simulink model "CryoDet6"  (R2015a)
settings: Solver=ode45  SolverMode=SingleTasking  StartTime=0.0  StopTime=1e-3  MaxStep=Tclk/8  RelTol=1e-3
values from neighbouring files (symbols this model uses):
  Fclk = Fadc/2    (= 185000000)    [setupCryoFPGA.m]    (also in setupCryoNew.m)
  noise = exp(1i*phi)    [setupCryoFPGA.m]    (also in setupCryoNew.m = exp(2i*pi*rand(1, noiseLen)))
  noiseLen = 128    [setupCryoFPGA.m]    (also in setupCryoNew.m)
  noiseSteps = 32    [setupCryoFPGA.m]    (also in setupCryoNew.m)
  notch = tf( [1 a*wNotch/Q wNotch^2], [1 wNotch/Q wNotch^2])    [setupCryoFPGA.m]    (also in setupCryoNew.m)
  notch2 = tf( [1 a*wNotch/Q wNotch^2], [1 wNotch/Q wNotch^2])    [setupCryoFPGA.m]    (also in setupCryoNew.m)
  setupVers = 5    [setupCryoFPGA.m]    (also in setupCryoNew.m = 21)
  Tclk = 1/Fclk    (= 5.40540540541e-09)    [setupCryoFPGA.m]    (also in setupCryoNew.m)
  wTs1 = w1*Ts1    (= 0.0271705310581)    [setupCryoFPGA.m]
undefined symbols (not defined in the file or in its folder): AXI4, Lite, xlipgetpartsetting
libraries: xbsIndex_r4 x516, simulink x1
(part 1 of 6)
settings Model: CovSFcnEnable=off  Creator=ssmith  LastModifiedBy=ssmith
settings OptimizationCC: BlockReduction=off  BooleanDataType=off
settings DebuggingCC: SaveWithParameterizedLinksMsg=none  UnderspecifiedInitializationDetection=Classic  MergeDetectMultiDrivingBlocksExec=none  SignalResolutionControl=TryResolveAllWithWarning
settings HardwareCC: TargetUnknown=on

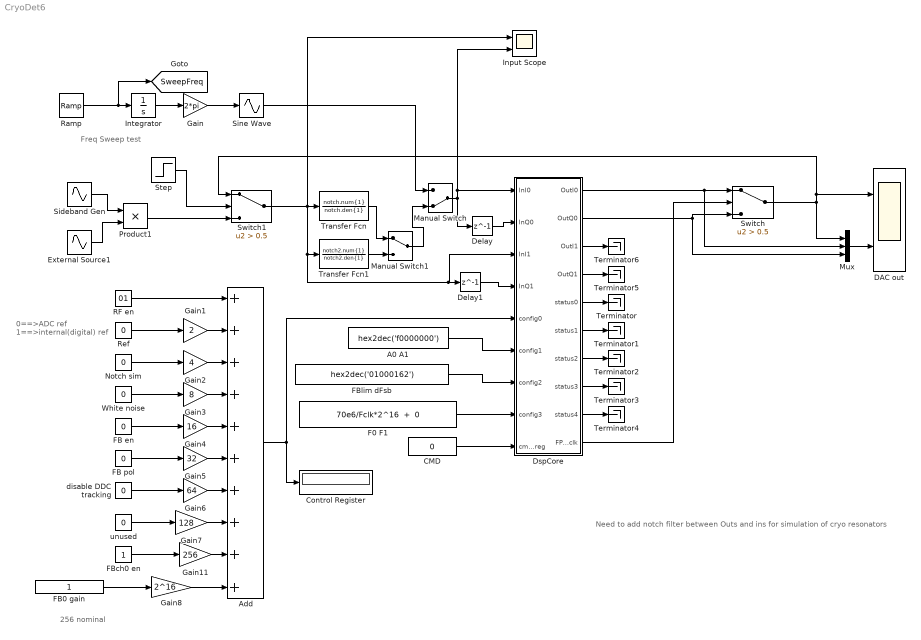
== system CryoDet6 ==
  note: 256 nominal
  note: 0==>ADC ref
      | 1==>internal(digital) ref
  note: Freq Sweep test
  note: Need to add notch filter between Outs and ins for simulation of cryo resonators
  A0 A1 : Constant  Value=hex2dec('f0000000')  SampleTime=Tclk
  Add : Sum  Inputs=++++++++++
  CMD : Constant  Value=0  SampleTime=Tclk
  Control Register : Display
      settings: Format=hex (Stored Integer)  Decimation=1000
  DAC out : Scope  NumInputPorts=2
      settings: TickLabels=on  TimeRange=3.316216230427035e-06  YMin=-1~-1  YMax=1~1  SaveName=DACscope  SampleTime=0.1e-6
  Delay : Delay  DelayLength=1  SampleTime=Tclk/2
  Delay1 : Delay  DelayLength=1  SampleTime=Tclk/2
  DspCore : Subsystem
  External Source1 : Sin  Amplitude=.8  Frequency=2*pi*70e6  SampleTime=0
  F0 F1 : Constant  Value="70e6/Fclk*2^16  +  0"  SampleTime=Tclk
  FB en : Constant  Value=0  SampleTime=Tclk
  FB pol : Constant  Value=0  SampleTime=Tclk
  FB0 gain : Constant  SampleTime=Tclk
  FBch0 en : Constant  SampleTime=Tclk
  FBlim dFsb : Constant  Value=hex2dec('01000162')  SampleTime=Tclk
  Gain : Gain  Gain=2*pi
  Gain1 : Gain  Gain=2
  Gain11 : Gain  Gain=256
  Gain2 : Gain  Gain=4
  Gain3 : Gain  Gain=8
  Gain4 : Gain  Gain=16
  Gain5 : Gain  Gain=32
  Gain6 : Gain  Gain=64
  Gain7 : Gain  Gain=128
  Gain8 : Gain  Gain=2^16
  Input Scope : Scope  NumInputPorts=2
      settings: TimeRange=6.755405405405412e-06  YMin=-1~-5e-147  YMax=1~5e-147  SaveName=ScopeData18
  Integrator : Integrator
  Manual Switch : ManualSwitch  CurrentSetting=0
  Manual Switch1 : ManualSwitch
  Mux : Mux  Inputs=3
  Notch sim : Constant  Value=0  SampleTime=Tclk
  Product1 : Product
  RF en : Constant  Value=01  SampleTime=Tclk
  Ramp : simulink/Sources/Ramp  slope=0.4e6/1e-3  start=0  X0=69.8e6
  Ref : Constant  Value=0  SampleTime=Tclk
  Sideband Gen : Sin  Amplitude=0.18  Bias=0.8  Frequency=2*pi*1e6  SampleTime=0
  Sine Wave : Sin  TimeSource=Use external signal  SampleTime=0
  Step : Step  Time=1e-6  SampleTime=0
  Switch : Switch  Criteria=u2 > Threshold  Threshold=0.5
  Switch1 : Switch  Criteria=u2 > Threshold  Threshold=0.5
  Terminator{,1..6} (7 alike) : Terminator
  Transfer Fcn : TransferFcn  Numerator=notch.num{1}  Denominator=notch.den{1}
  Transfer Fcn1 : TransferFcn  Numerator=notch2.num{1}  Denominator=notch2.den{1}
  White noise : Constant  Value=0  SampleTime=Tclk
  disable DDC tracking : Constant  Value=0  SampleTime=Tclk
  unused : Constant  Value=0  SampleTime=Tclk
  tag scope: SweepFreq=global
  wires:
  Add/1 -> DspCore/5(config0), Control Register/1
  A0 A1/1 -> DspCore/6(config1)
  FBlim dFsb/1 -> DspCore/7(config2)
  F0 F1/1 -> DspCore/8(config3)
  CMD/1 -> DspCore/9(cmd_reg)
  Delay/1 -> DspCore/2(InQ0)
  Delay1/1 -> DspCore/4(InQ1)
  DspCore/5(status0) -> Terminator/1
  DspCore/6(status1) -> Terminator1/1
  DspCore/7(status2) -> Terminator2/1
  DspCore/8(status3) -> Terminator3/1
  DspCore/9(status4) -> Terminator4/1
  Sideband Gen/1 -> Product1/1
  DspCore/10(FPGAclk) -> Switch/2
  DspCore/2(OutQ0) -> Mux/3, Switch/3
  Switch/1 -> DAC out/1, Switch1/1, Mux/1
  DspCore/1(OutI0) -> Switch/1, Mux/2
  Product1/1 -> Switch1/3
  Step/1 -> Switch1/2
  Manual Switch/1 -> Input Scope/2, DspCore/1(InI0), Delay/1
  Sine Wave/1 -> Manual Switch/1
  Ramp/1 -> [SweepFreq], Integrator/1
  Gain/1 -> Sine Wave/1
  Integrator/1 -> Gain/1
  Switch1/1 -> Transfer Fcn1/1, DspCore/3(InI1), Delay1/1, Input Scope/1, Transfer Fcn/1
  External Source1/1 -> Product1/2
  Transfer Fcn1/1 -> Manual Switch1/2
  Transfer Fcn/1 -> Manual Switch1/1
  Manual Switch1/1 -> Manual Switch/2
  RF en/1 -> Add/1
  Ref/1 -> Gain1/1
  Notch sim/1 -> Gain2/1
  White noise/1 -> Gain3/1
  FB en/1 -> Gain4/1
  FB pol/1 -> Gain5/1
  disable DDC tracking/1 -> Gain6/1
  unused/1 -> Gain7/1
  Gain1/1 -> Add/2
  Gain2/1 -> Add/3
  Gain3/1 -> Add/4
  Gain4/1 -> Add/5
  Gain5/1 -> Add/6
  Gain6/1 -> Add/7
  Gain7/1 -> Add/8
  FBch0 en/1 -> Gain11/1
  Gain11/1 -> Add/9
  Gain8/1 -> Add/10
  FB0 gain/1 -> Gain8/1
  DspCore/3(OutI1) -> Terminator6/1
  DspCore/4(OutQ1) -> Terminator5/1
  Mux/1 -> DAC out/2

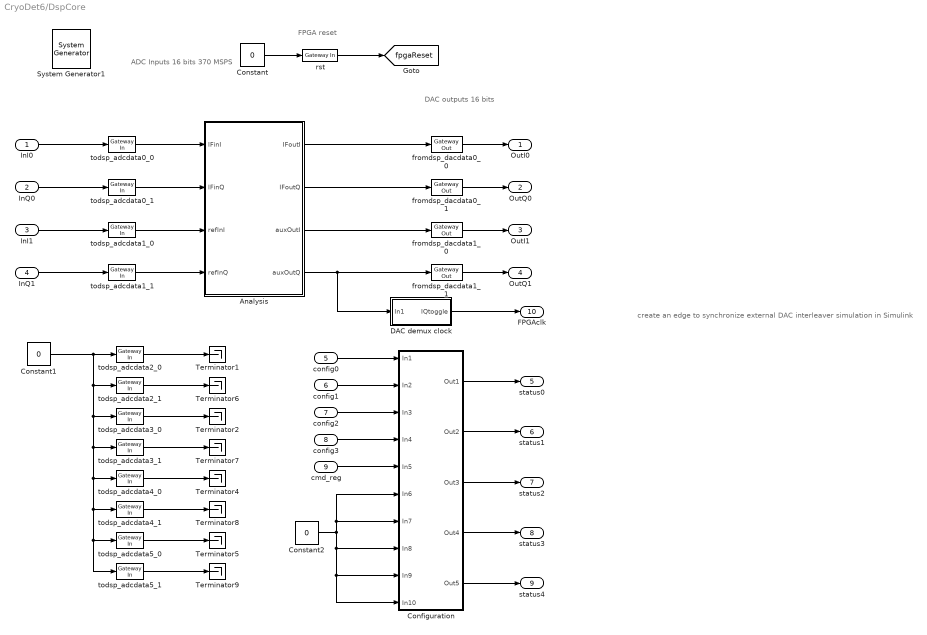
== system CryoDet6/DspCore ==
  note: create an edge to synchronize external DAC interleaver simulation in Simulink
  note: DAC outputs
      | 16 bits
  note: ADC Inputs
      | 16 bits
      | 370 MSPS
  note: FPGA reset
  InI0 : Inport
  InQ0 : Inport  Port=2
  InI1 : Inport  Port=3
  InQ1 : Inport  Port=4
  config0 : Inport  Port=5
  config1 : Inport  Port=6
  config2 : Inport  Port=7
  config3 : Inport  Port=8
  cmd_reg : Inport  Port=9
  " System Generator1" : xbsIndex_r4/ System Generator  Tag=genX  xilinxfamily=kintexu  part=xcku040  speed=-2-e  package=ffva1156  synthesis_tool=Vivado  clock_wrapper=Clock Enables  directory=./netlist  proj_type=Vivado  Synth_file=Vivado Synthesis Defaults  Impl_file=Vivado Implementation Defaults  testbench=off  simulink_period=Tclk  sysclk_period=Tclk*1e9  dcm_input_clock_period=10  incr_netlist=off  trim_vbits=Everywhere in SubSystem  dbl_ovrd=According to Block Masks  core_generation=According to Block Masks  run_coregen=off  deprecated_control=off  eval_field=0  block_type=sysgen
  Analysis : Subsystem
  Configuration : Subsystem
  Constant : Constant  Value=0
  Constant1 : Constant  Value=0
  Constant2 : Constant  Value=0
  DAC demux clock : Subsystem
  Terminator{1..2,4..9} (8 alike) : Terminator
  fromdsp_dacdata0_0 : xbsIndex_r4/Gateway Out  inherit_from_input=on  hdl_port=on  rows=1  columns=1  UseAsDAC=off  DACChannel='1'  interface=None  automatic_assignment=on  address_offset=hex2dec('00')  intf_name=''  intf_description=''  timing_constraint=None  locs_specified=off  LOCs={}  io_standard={}  block_type=gatewayout
  fromdsp_dacdata0_1 : xbsIndex_r4/Gateway Out  inherit_from_input=on  hdl_port=on  rows=1  columns=1  UseAsDAC=off  DACChannel='1'  interface=None  automatic_assignment=on  address_offset=hex2dec('00')  intf_name=''  intf_description=''  timing_constraint=None  locs_specified=off  LOCs={}  io_standard={}  block_type=gatewayout
  fromdsp_dacdata1_0 : xbsIndex_r4/Gateway Out  inherit_from_input=on  hdl_port=on  rows=1  columns=1  UseAsDAC=off  DACChannel='1'  interface=None  automatic_assignment=on  address_offset=hex2dec('00')  intf_name=''  intf_description=''  timing_constraint=None  locs_specified=off  LOCs={}  io_standard={}  block_type=gatewayout
  fromdsp_dacdata1_1 : xbsIndex_r4/Gateway Out  inherit_from_input=off  hdl_port=on  rows=1  columns=1  UseAsDAC=off  DACChannel='1'  interface=None  automatic_assignment=on  address_offset=hex2dec('00')  intf_name=''  intf_description=''  timing_constraint=None  locs_specified=off  LOCs={}  io_standard={}  block_type=gatewayout
  rst : xbsIndex_r4/Gateway In  gui_display_data_type=Boolean  arith_type=Boolean  n_bits=16  bin_pt=14  preci_type=Single  exp_width=8  frac_width=24  rows=1  columns=1  quantization="Round  (unbiased: +/- Inf)"  overflow=Saturate  period=Tclk  UseAsADC=off  ADCChannel='1'  interface=None  automatic_assignment=on  address_offset=hex2dec('00')  intf_name=''  intf_description=''  timing_constraint=None  locs_specified=off  LOCs={}  io_standard={}  inherit_from_input=off  hdl_port=on  dbl_ovrd=off  block_type=gatewayin
  todsp_adcdata0_0 : xbsIndex_r4/Gateway In  gui_display_data_type=Fixed-point  arith_type="Signed  (2's comp)"  n_bits=16  bin_pt=15  preci_type=Single  exp_width=8  frac_width=24  rows=1  columns=1  quantization=Truncate  overflow=Wrap  period=Tclk  UseAsADC=off  ADCChannel='1'  interface=None  automatic_assignment=on  address_offset=hex2dec('00')  intf_name=''  intf_description=''  timing_constraint=None  locs_specified=off  LOCs={}  io_standard={}  inherit_from_input=off  hdl_port=on  dbl_ovrd=off  block_type=gatewayin
  todsp_adcdata0_1 : xbsIndex_r4/Gateway In  gui_display_data_type=Fixed-point  arith_type="Signed  (2's comp)"  n_bits=16  bin_pt=15  preci_type=Single  exp_width=8  frac_width=24  rows=1  columns=1  quantization=Truncate  overflow=Wrap  period=Tclk  UseAsADC=off  ADCChannel='1'  interface=None  automatic_assignment=on  address_offset=hex2dec('00')  intf_name=''  intf_description=''  timing_constraint=None  locs_specified=off  LOCs={}  io_standard={}  inherit_from_input=off  hdl_port=on  dbl_ovrd=off  block_type=gatewayin
  todsp_adcdata1_0 : xbsIndex_r4/Gateway In  gui_display_data_type=Fixed-point  arith_type="Signed  (2's comp)"  n_bits=16  bin_pt=15  preci_type=Single  exp_width=8  frac_width=24  rows=1  columns=1  quantization=Truncate  overflow=Wrap  period=Tclk  UseAsADC=off  ADCChannel='1'  interface=None  automatic_assignment=on  address_offset=hex2dec('00')  intf_name=''  intf_description=''  timing_constraint=None  locs_specified=off  LOCs={}  io_standard={}  inherit_from_input=off  hdl_port=on  dbl_ovrd=off  block_type=gatewayin
  todsp_adcdata1_1 : xbsIndex_r4/Gateway In  gui_display_data_type=Fixed-point  arith_type="Signed  (2's comp)"  n_bits=16  bin_pt=15  preci_type=Single  exp_width=8  frac_width=24  rows=1  columns=1  quantization=Truncate  overflow=Wrap  period=Tclk  UseAsADC=off  ADCChannel='1'  interface=None  automatic_assignment=on  address_offset=hex2dec('00')  intf_name=''  intf_description=''  timing_constraint=None  locs_specified=off  LOCs={}  io_standard={}  inherit_from_input=off  hdl_port=on  dbl_ovrd=off  block_type=gatewayin
  todsp_adcdata2_0 : xbsIndex_r4/Gateway In  gui_display_data_type=Fixed-point  arith_type="Signed  (2's comp)"  n_bits=16  bin_pt=15  preci_type=Single  exp_width=8  frac_width=24  rows=1  columns=1  quantization=Truncate  overflow=Wrap  period=Tclk  UseAsADC=off  ADCChannel='1'  interface=None  automatic_assignment=on  address_offset=hex2dec('00')  intf_name=''  intf_description=''  timing_constraint=None  locs_specified=off  LOCs={}  io_standard={}  inherit_from_input=off  hdl_port=on  dbl_ovrd=off  block_type=gatewayin
  todsp_adcdata2_1 : xbsIndex_r4/Gateway In  gui_display_data_type=Fixed-point  arith_type="Signed  (2's comp)"  n_bits=16  bin_pt=15  preci_type=Single  exp_width=8  frac_width=24  rows=1  columns=1  quantization=Truncate  overflow=Wrap  period=Tclk  UseAsADC=off  ADCChannel='1'  interface=None  automatic_assignment=on  address_offset=hex2dec('00')  intf_name=''  intf_description=''  timing_constraint=None  locs_specified=off  LOCs={}  io_standard={}  inherit_from_input=off  hdl_port=on  dbl_ovrd=off  block_type=gatewayin
  todsp_adcdata3_0 : xbsIndex_r4/Gateway In  gui_display_data_type=Fixed-point  arith_type="Signed  (2's comp)"  n_bits=16  bin_pt=15  preci_type=Single  exp_width=8  frac_width=24  rows=1  columns=1  quantization=Truncate  overflow=Wrap  period=Tclk  UseAsADC=off  ADCChannel='1'  interface=None  automatic_assignment=on  address_offset=hex2dec('00')  intf_name=''  intf_description=''  timing_constraint=None  locs_specified=off  LOCs={}  io_standard={}  inherit_from_input=off  hdl_port=on  dbl_ovrd=off  block_type=gatewayin
  todsp_adcdata3_1 : xbsIndex_r4/Gateway In  gui_display_data_type=Fixed-point  arith_type="Signed  (2's comp)"  n_bits=16  bin_pt=15  preci_type=Single  exp_width=8  frac_width=24  rows=1  columns=1  quantization=Truncate  overflow=Wrap  period=Tclk  UseAsADC=off  ADCChannel='1'  interface=None  automatic_assignment=on  address_offset=hex2dec('00')  intf_name=''  intf_description=''  timing_constraint=None  locs_specified=off  LOCs={}  io_standard={}  inherit_from_input=off  hdl_port=on  dbl_ovrd=off  block_type=gatewayin
  todsp_adcdata4_0 : xbsIndex_r4/Gateway In  gui_display_data_type=Fixed-point  arith_type="Signed  (2's comp)"  n_bits=16  bin_pt=15  preci_type=Single  exp_width=8  frac_width=24  rows=1  columns=1  quantization=Truncate  overflow=Wrap  period=Tclk  UseAsADC=off  ADCChannel='1'  interface=None  automatic_assignment=on  address_offset=hex2dec('00')  intf_name=''  intf_description=''  timing_constraint=None  locs_specified=off  LOCs={}  io_standard={}  inherit_from_input=off  hdl_port=on  dbl_ovrd=off  block_type=gatewayin
  todsp_adcdata4_1 : xbsIndex_r4/Gateway In  gui_display_data_type=Fixed-point  arith_type="Signed  (2's comp)"  n_bits=16  bin_pt=15  preci_type=Single  exp_width=8  frac_width=24  rows=1  columns=1  quantization=Truncate  overflow=Wrap  period=Tclk  UseAsADC=off  ADCChannel='1'  interface=None  automatic_assignment=on  address_offset=hex2dec('00')  intf_name=''  intf_description=''  timing_constraint=None  locs_specified=off  LOCs={}  io_standard={}  inherit_from_input=off  hdl_port=on  dbl_ovrd=off  block_type=gatewayin
  todsp_adcdata5_0 : xbsIndex_r4/Gateway In  gui_display_data_type=Fixed-point  arith_type="Signed  (2's comp)"  n_bits=16  bin_pt=15  preci_type=Single  exp_width=8  frac_width=24  rows=1  columns=1  quantization=Truncate  overflow=Wrap  period=Tclk  UseAsADC=off  ADCChannel='1'  interface=None  automatic_assignment=on  address_offset=hex2dec('00')  intf_name=''  intf_description=''  timing_constraint=None  locs_specified=off  LOCs={}  io_standard={}  inherit_from_input=off  hdl_port=on  dbl_ovrd=off  block_type=gatewayin
  todsp_adcdata5_1 : xbsIndex_r4/Gateway In  gui_display_data_type=Fixed-point  arith_type="Signed  (2's comp)"  n_bits=16  bin_pt=15  preci_type=Single  exp_width=8  frac_width=24  rows=1  columns=1  quantization=Truncate  overflow=Wrap  period=Tclk  UseAsADC=off  ADCChannel='1'  interface=None  automatic_assignment=on  address_offset=hex2dec('00')  intf_name=''  intf_description=''  timing_constraint=None  locs_specified=off  LOCs={}  io_standard={}  inherit_from_input=off  hdl_port=on  dbl_ovrd=off  block_type=gatewayin
  OutI0 : Outport
  OutQ0 : Outport  Port=2
  OutI1 : Outport  Port=3
  OutQ1 : Outport  Port=4
  status0 : Outport  Port=5
  status1 : Outport  Port=6
  status2 : Outport  Port=7
  status3 : Outport  Port=8
  status4 : Outport  Port=9
  FPGAclk : Outport  Port=10
  tag scope: fpgaReset=global
  wires:
  InI0/1 -> todsp_adcdata0_0/1
  fromdsp_dacdata1_0/1 -> OutI1/1
  fromdsp_dacdata0_0/1 -> OutI0/1
  todsp_adcdata0_0/1 -> Analysis/1(IFinI)
  InI1/1 -> todsp_adcdata1_0/1
  Constant/1 -> rst/1
  rst/1 -> [fpgaReset]
  todsp_adcdata2_0/1 -> Terminator1/1
  todsp_adcdata3_0/1 -> Terminator2/1
  todsp_adcdata4_0/1 -> Terminator4/1
  todsp_adcdata5_0/1 -> Terminator5/1
  InQ0/1 -> todsp_adcdata0_1/1
  todsp_adcdata0_1/1 -> Analysis/2(IFinQ)
  fromdsp_dacdata0_1/1 -> OutQ0/1
  fromdsp_dacdata1_1/1 -> OutQ1/1
  InQ1/1 -> todsp_adcdata1_1/1
  todsp_adcdata2_1/1 -> Terminator6/1
  todsp_adcdata3_1/1 -> Terminator7/1
  todsp_adcdata4_1/1 -> Terminator8/1
  todsp_adcdata5_1/1 -> Terminator9/1
  Analysis/1(IFoutI) -> fromdsp_dacdata0_0/1
  Analysis/2(IFoutQ) -> fromdsp_dacdata0_1/1
  config0/1 -> Configuration/1(In1)
  config1/1 -> Configuration/2(In2)
  config2/1 -> Configuration/3(In3)
  config3/1 -> Configuration/4(In4)
  cmd_reg/1 -> Configuration/5(In5)
  Configuration/1(Out1) -> status0/1
  Configuration/2(Out2) -> status1/1
  Configuration/3(Out3) -> status2/1
  Configuration/4(Out4) -> status3/1
  Configuration/5(Out5) -> status4/1
  Analysis/3(auxOutI) -> fromdsp_dacdata1_0/1
  Analysis/4(auxOutQ) -> DAC demux clock/1(In1), fromdsp_dacdata1_1/1
  todsp_adcdata1_0/1 -> Analysis/3(refInI)
  todsp_adcdata1_1/1 -> Analysis/4(refInQ)
  Constant1/1 -> todsp_adcdata3_0/1, todsp_adcdata3_1/1, todsp_adcdata4_1/1, todsp_adcdata5_0/1, todsp_adcdata5_1/1, todsp_adcdata4_0/1, todsp_adcdata2_1/1, todsp_adcdata2_0/1
  Constant2/1 -> Configuration/10(In10), Configuration/9(In9), Configuration/8(In8), Configuration/7(In7), Configuration/6(In6)
  DAC demux clock/1(IQtoggle) -> FPGAclk/1

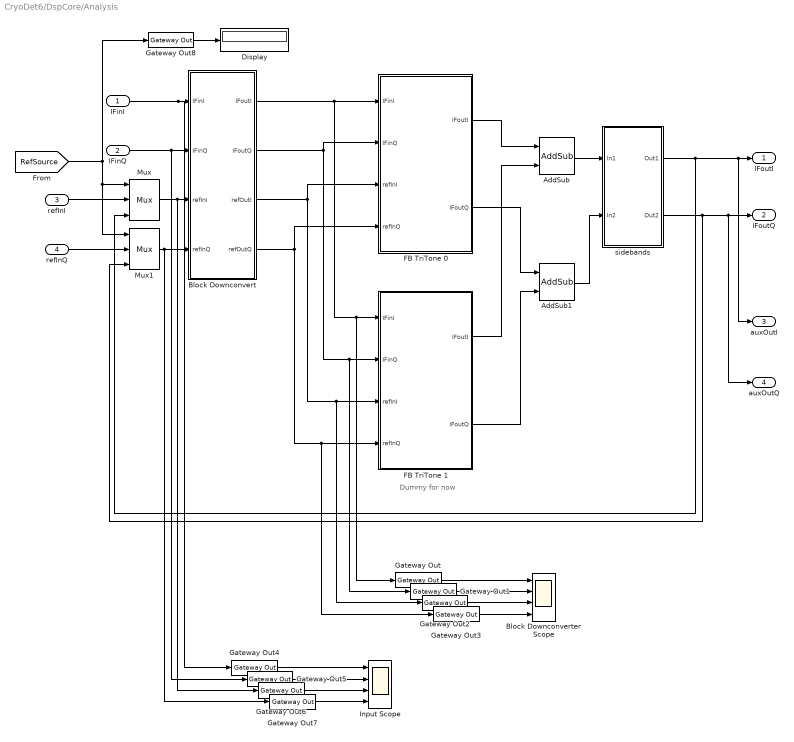
== system CryoDet6/DspCore/Analysis ==
  note: Dummy for now
  IFinI : Inport
  IFinQ : Inport  Port=2
  refInI : Inport  Port=3
  refInQ : Inport  Port=4
  AddSub : xbsIndex_r4/AddSub  mode=Addition  use_carryin=off  use_carryout=off  en=off  latency=3  precision=User Defined  arith_type="Signed  (2's comp)"  n_bits=16  bin_pt=15  quantization=Truncate  overflow=Saturate  use_behavioral_HDL=off  hw_selection=Fabric  pipelined=off  dbl_ovrd=off  block_type=addsub
  AddSub1 : xbsIndex_r4/AddSub  mode=Addition  use_carryin=off  use_carryout=off  en=off  latency=3  precision=User Defined  arith_type="Signed  (2's comp)"  n_bits=16  bin_pt=15  quantization=Truncate  overflow=Saturate  use_behavioral_HDL=off  hw_selection=Fabric  pipelined=off  dbl_ovrd=off  block_type=addsub
  Block Downconverter Scope : Scope  NumInputPorts=4
      settings: TimeRange=1e-05  YMin=-1~-1~-0.75~-0.75  YMax=1~1~0.75~0.75  SaveName=ScopeData3
  Block Downconvert : Subsystem
  Display : Display
  FB TriTone 0 : Subsystem
  FB TriTone 1 : Subsystem
  Gateway Out{,1..8} (9 alike) : xbsIndex_r4/Gateway Out  inherit_from_input=off  hdl_port=off  rows=1  columns=1  UseAsDAC=off  DACChannel='1'  interface=None  automatic_assignment=on  address_offset=hex2dec('00')  intf_name=''  intf_description=''  timing_constraint=None  locs_specified=off  LOCs={}  io_standard={}  block_type=gatewayout
  Input Scope : Scope  NumInputPorts=4
      settings: TimeRange=2e-06  YMin=-1~-1~-1~-1  YMax=1~1~1~1  SaveName=ScopeData5
  Mux : xbsIndex_r4/Mux  inputs=2  en=off  latency=1  precision=Full  arith_type=Unsigned  n_bits=16  bin_pt=14  quantization=Truncate  overflow=Wrap  dbl_ovrd=off  block_type=mux
  Mux1 : xbsIndex_r4/Mux  inputs=2  en=off  latency=1  precision=Full  arith_type=Unsigned  n_bits=16  bin_pt=14  quantization=Truncate  overflow=Wrap  dbl_ovrd=off  block_type=mux
  sidebands : Subsystem
  IFoutI : Outport
  IFoutQ : Outport  Port=2
  auxOutI : Outport  Port=3
  auxOutQ : Outport  Port=4
  wires:
  IFinI/1 -> Gateway Out4/1, Block Downconvert/1(IFinI)
  IFinQ/1 -> Gateway Out5/1, Block Downconvert/2(IFinQ)
  sidebands/1(Out1) -> Mux/3, auxOutI/1, IFoutI/1
  sidebands/2(Out2) -> Mux1/3, auxOutQ/1, IFoutQ/1
  Block Downconvert/1(IFoutI) -> Gateway Out/1, FB TriTone 1/1(IFinI), FB TriTone 0/1(IFinI)
  Block Downconvert/2(IFoutQ) -> Gateway Out1/1, FB TriTone 1/2(IFinQ), FB TriTone 0/2(IFinQ)
  Block Downconvert/3(refOutI) -> Gateway Out2/1, FB TriTone 1/3(refInI), FB TriTone 0/3(refInI)
  Block Downconvert/4(refOutQ) -> Gateway Out3/1, FB TriTone 1/4(refInQ), FB TriTone 0/4(refInQ)
  AddSub/1 -> sidebands/1(In1)
  FB TriTone 0/1(IFoutI) -> AddSub/1
  FB TriTone 1/1(IFoutI) -> AddSub/2
  AddSub1/1 -> sidebands/2(In2)
  FB TriTone 0/2(IFoutQ) -> AddSub1/1
  FB TriTone 1/2(IFoutQ) -> AddSub1/2
  [RefSource] -> Mux1/1, Mux/1, Gateway Out8/1
  refInI/1 -> Mux/2
  refInQ/1 -> Mux1/2
  Gateway Out/1 -> Block Downconverter Scope/1
  Gateway Out1/1 -> Block Downconverter Scope/2
  Gateway Out2/1 -> Block Downconverter Scope/3
  Gateway Out3/1 -> Block Downconverter Scope/4
  Mux/1 -> Gateway Out6/1, Block Downconvert/3(refInI)
  Mux1/1 -> Gateway Out7/1, Block Downconvert/4(refInQ)
  Gateway Out4/1 -> Input Scope/1
  Gateway Out5/1 -> Input Scope/2
  Gateway Out6/1 -> Input Scope/3
  Gateway Out7/1 -> Input Scope/4
  Gateway Out8/1 -> Display/1

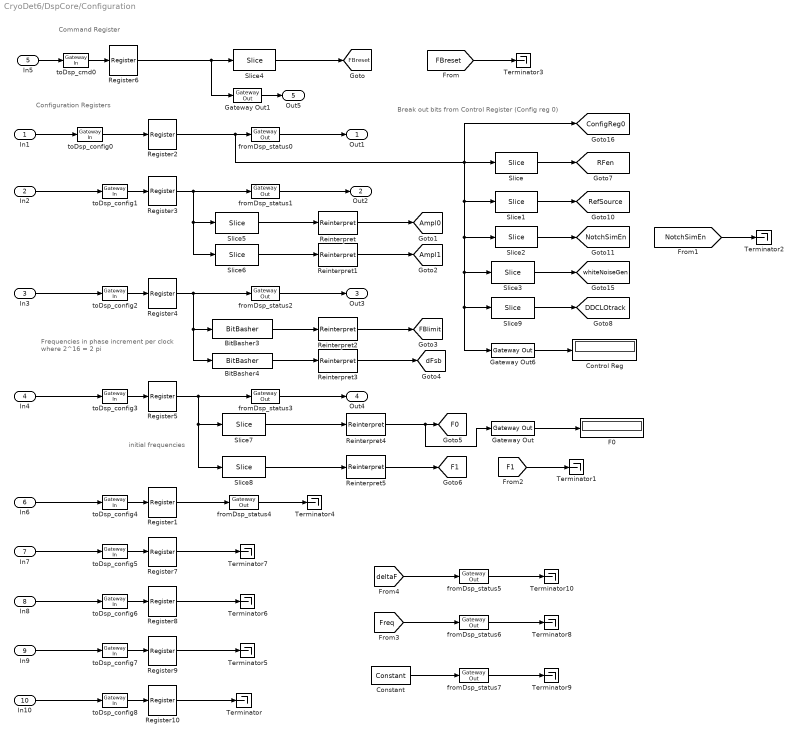
== system CryoDet6/DspCore/Configuration ==
  note: Frequencies in phase increment per clock
      | where 2^16 = 2 pi
  note: initial frequencies
  note: Configuration Registers
  note: Command Register
  note: Break out bits from Control Register (Config reg 0)
  In1 : Inport
  In2 : Inport  Port=2
  In3 : Inport  Port=3
  In4 : Inport  Port=4
  In5 : Inport  Port=5
  In6 : Inport  Port=6
  In7 : Inport  Port=7
  In8 : Inport  Port=8
  In9 : Inport  Port=9
  In10 : Inport  Port=10
  BitBasher3 : xbsIndex_r4/BitBasher  bitexpr=a={b[31:16]}  display_expr=on  sr_1=a  arith_type1=Unsigned  bin_pt1=0  sr_2=2  arith_type2=Unsigned  bin_pt2=0  sr_3=3  arith_type3=Unsigned  bin_pt3=0  sr_4=4  arith_type4=Unsigned  bin_pt4=0  dbl_ovrd=off  block_type=bitbasher
  BitBasher4 : xbsIndex_r4/BitBasher  bitexpr=a={b[15:0]}  display_expr=on  sr_1=a  arith_type1=Unsigned  bin_pt1=16  sr_2=2  arith_type2=Unsigned  bin_pt2=0  sr_3=3  arith_type3=Unsigned  bin_pt3=0  sr_4=4  arith_type4=Unsigned  bin_pt4=0  dbl_ovrd=off  block_type=bitbasher
  Constant : xbsIndex_r4/Constant  const=setupVers  gui_display_data_type=Fixed-point  arith_type=Signed (2's comp)  n_bits=32  bin_pt=0  preci_type=Single  exp_width=8  frac_width=24  explicit_period=off  period=1  equ=P=C  opselect=C  inp2=PCIN>>17  opr=+  inp1=P  carry=CIN  dbl_ovrd=off  block_type=constant
  Control Reg : Display
  F0 : Display
  Gateway Out : xbsIndex_r4/Gateway Out  inherit_from_input=on  hdl_port=off  rows=1  columns=1  UseAsDAC=off  DACChannel='1'  interface=None  automatic_assignment=on  address_offset=hex2dec('00')  intf_name=''  intf_description=''  timing_constraint=None  locs_specified=off  LOCs={}  io_standard={}  block_type=gatewayout
  Gateway Out1 : xbsIndex_r4/Gateway Out  inherit_from_input=off  hdl_port=off  rows=1  columns=1  UseAsDAC=off  DACChannel='1'  interface=None  automatic_assignment=on  address_offset=hex2dec('00')  intf_name=''  intf_description=''  timing_constraint=None  locs_specified=off  LOCs={}  io_standard={}  block_type=gatewayout
  Gateway Out6 : xbsIndex_r4/Gateway Out  inherit_from_input=off  hdl_port=off  rows=1  columns=1  UseAsDAC=off  DACChannel='1'  interface=None  automatic_assignment=on  address_offset=hex2dec('00')  intf_name=''  intf_description=''  timing_constraint=None  locs_specified=off  LOCs={}  io_standard={}  block_type=gatewayout
  Register{1..10} (10 alike) : xbsIndex_r4/Register  init=0  rst=off  en=off  dbl_ovrd=off  block_type=register
  Reinterpret : xbsIndex_r4/Reinterpret  force_arith_type=on  arith_type=Unsigned  force_bin_pt=on  bin_pt=16  block_type=reinterpret
  Reinterpret1 : xbsIndex_r4/Reinterpret  force_arith_type=on  arith_type=Unsigned  force_bin_pt=on  bin_pt=16  block_type=reinterpret
  Reinterpret2 : xbsIndex_r4/Reinterpret  force_arith_type=on  arith_type="Signed  (2's comp)"  force_bin_pt=on  bin_pt=16  block_type=reinterpret
  Reinterpret3 : xbsIndex_r4/Reinterpret  force_arith_type=on  arith_type=Unsigned  force_bin_pt=on  bin_pt=16  block_type=reinterpret
  Reinterpret4 : xbsIndex_r4/Reinterpret  force_arith_type=on  arith_type="Signed  (2's comp)"  force_bin_pt=on  bin_pt=16  block_type=reinterpret
  Reinterpret5 : xbsIndex_r4/Reinterpret  force_arith_type=on  arith_type="Signed  (2's comp)"  force_bin_pt=on  bin_pt=16  block_type=reinterpret
  Slice : xbsIndex_r4/Slice  nbits=1  boolean_output=on  mode=Upper Bit Location + Width  bit1=0  base1=LSB of Input  bit0=0  base0=LSB of Input  dbl_ovrd=off  block_type=slice
  Slice1 : xbsIndex_r4/Slice  nbits=1  boolean_output=on  mode=Upper Bit Location + Width  bit1=1  base1=LSB of Input  bit0=0  base0=LSB of Input  dbl_ovrd=off  block_type=slice
  Slice2 : xbsIndex_r4/Slice  nbits=1  boolean_output=on  mode=Upper Bit Location + Width  bit1=2  base1=LSB of Input  bit0=0  base0=LSB of Input  dbl_ovrd=off  block_type=slice
  Slice3 : xbsIndex_r4/Slice  nbits=1  boolean_output=on  mode=Upper Bit Location + Width  bit1=3  base1=LSB of Input  bit0=0  base0=LSB of Input  dbl_ovrd=off  block_type=slice
  Slice4 : xbsIndex_r4/Slice  nbits=1  boolean_output=on  mode=Upper Bit Location + Width  bit1=0  base1=LSB of Input  bit0=0  base0=LSB of Input  dbl_ovrd=off  block_type=slice
  Slice5 : xbsIndex_r4/Slice  nbits=16  boolean_output=off  mode=Upper Bit Location + Width  bit1=31  base1=LSB of Input  bit0=0  base0=LSB of Input  dbl_ovrd=off  block_type=slice
  Slice6 : xbsIndex_r4/Slice  nbits=16  boolean_output=off  mode=Upper Bit Location + Width  bit1=15  base1=LSB of Input  bit0=0  base0=LSB of Input  dbl_ovrd=off  block_type=slice
  Slice7 : xbsIndex_r4/Slice  nbits=16  boolean_output=off  mode=Upper Bit Location + Width  bit1=15  base1=LSB of Input  bit0=0  base0=LSB of Input  dbl_ovrd=off  block_type=slice
  Slice8 : xbsIndex_r4/Slice  nbits=16  boolean_output=off  mode=Upper Bit Location + Width  bit1=31  base1=LSB of Input  bit0=0  base0=LSB of Input  dbl_ovrd=off  block_type=slice
  Slice9 : xbsIndex_r4/Slice  nbits=1  boolean_output=on  mode=Upper Bit Location + Width  bit1=6  base1=LSB of Input  bit0=0  base0=LSB of Input  dbl_ovrd=off  block_type=slice
  Terminator{,1..10} (11 alike) : Terminator
  fromDsp_status0 : xbsIndex_r4/Gateway Out  inherit_from_input=on  hdl_port=on  rows=1  columns=1  UseAsDAC=off  DACChannel='1'  interface=AXI4-Lite  automatic_assignment=off  address_offset=hex2dec('00')  intf_name=''  intf_description=''  timing_constraint=None  locs_specified=off  LOCs={}  io_standard={}  block_type=gatewayout
  fromDsp_status1 : xbsIndex_r4/Gateway Out  inherit_from_input=on  hdl_port=on  rows=1  columns=1  UseAsDAC=off  DACChannel='1'  interface=AXI4-Lite  automatic_assignment=off  address_offset=hex2dec('04')  intf_name=''  intf_description=''  timing_constraint=None  locs_specified=off  LOCs={}  io_standard={}  block_type=gatewayout
  fromDsp_status2 : xbsIndex_r4/Gateway Out  inherit_from_input=on  hdl_port=on  rows=1  columns=1  UseAsDAC=off  DACChannel='1'  interface=AXI4-Lite  automatic_assignment=off  address_offset=hex2dec('08')  intf_name=''  intf_description=''  timing_constraint=None  locs_specified=off  LOCs={}  io_standard={}  block_type=gatewayout
  fromDsp_status3 : xbsIndex_r4/Gateway Out  inherit_from_input=on  hdl_port=on  rows=1  columns=1  UseAsDAC=off  DACChannel='1'  interface=AXI4-Lite  automatic_assignment=off  address_offset=hex2dec('0C')  intf_name=''  intf_description=''  timing_constraint=None  locs_specified=off  LOCs={}  io_standard={}  block_type=gatewayout
  fromDsp_status4 : xbsIndex_r4/Gateway Out  inherit_from_input=on  hdl_port=on  rows=1  columns=1  UseAsDAC=off  DACChannel='1'  interface=AXI4-Lite  automatic_assignment=off  address_offset=hex2dec('10')  intf_name=''  intf_description=''  timing_constraint=None  locs_specified=off  LOCs={}  io_standard={}  block_type=gatewayout
  fromDsp_status5 : xbsIndex_r4/Gateway Out  inherit_from_input=on  hdl_port=on  rows=1  columns=1  UseAsDAC=off  DACChannel='1'  interface=AXI4-Lite  automatic_assignment=off  address_offset=hex2dec('14')  intf_name=''  intf_description=''  timing_constraint=None  locs_specified=off  LOCs={}  io_standard={}  block_type=gatewayout
  fromDsp_status6 : xbsIndex_r4/Gateway Out  inherit_from_input=on  hdl_port=on  rows=1  columns=1  UseAsDAC=off  DACChannel='1'  interface=AXI4-Lite  automatic_assignment=off  address_offset=hex2dec('18')  intf_name=''  intf_description=''  timing_constraint=None  locs_specified=off  LOCs={}  io_standard={}  block_type=gatewayout
  fromDsp_status7 : xbsIndex_r4/Gateway Out  inherit_from_input=on  hdl_port=on  rows=1  columns=1  UseAsDAC=off  DACChannel='1'  interface=AXI4-Lite  automatic_assignment=off  address_offset=hex2dec('1C')  intf_name=''  intf_description=''  timing_constraint=None  locs_specified=off  LOCs={}  io_standard={}  block_type=gatewayout
  toDsp_cmd0 : xbsIndex_r4/Gateway In  gui_display_data_type=Fixed-point  arith_type=Unsigned  n_bits=32  bin_pt=0  preci_type=Single  exp_width=8  frac_width=24  rows=1  columns=1  quantization=Truncate  overflow=Wrap  period=Tclk  UseAsADC=off  ADCChannel='1'  interface=AXI4-Lite  automatic_assignment=off  address_offset=hex2dec('90')  intf_name=''  intf_description=''  timing_constraint=None  locs_specified=off  LOCs={}  io_standard={}  inherit_from_input=off  hdl_port=on  dbl_ovrd=off  block_type=gatewayin
  toDsp_config0 : xbsIndex_r4/Gateway In  gui_display_data_type=Fixed-point  arith_type=Unsigned  n_bits=32  bin_pt=0  preci_type=Single  exp_width=8  frac_width=24  rows=1  columns=1  quantization=Truncate  overflow=Wrap  period=Tclk  UseAsADC=off  ADCChannel='1'  interface=AXI4-Lite  automatic_assignment=off  address_offset=hex2dec('80')  intf_name=''  intf_description=''  timing_constraint=None  locs_specified=off  LOCs={}  io_standard={}  inherit_from_input=off  hdl_port=on  dbl_ovrd=off  block_type=gatewayin
  toDsp_config1 : xbsIndex_r4/Gateway In  gui_display_data_type=Fixed-point  arith_type=Unsigned  n_bits=32  bin_pt=0  preci_type=Single  exp_width=8  frac_width=24  rows=1  columns=1  quantization=Truncate  overflow=Wrap  period=Tclk  UseAsADC=off  ADCChannel='1'  interface=AXI4-Lite  automatic_assignment=off  address_offset=hex2dec('84')  intf_name=''  intf_description=''  timing_constraint=None  locs_specified=off  LOCs={}  io_standard={}  inherit_from_input=off  hdl_port=on  dbl_ovrd=off  block_type=gatewayin
  toDsp_config2 : xbsIndex_r4/Gateway In  gui_display_data_type=Fixed-point  arith_type=Unsigned  n_bits=32  bin_pt=0  preci_type=Single  exp_width=8  frac_width=24  rows=1  columns=1  quantization=Truncate  overflow=Wrap  period=Tclk  UseAsADC=off  ADCChannel='1'  interface=AXI4-Lite  automatic_assignment=off  address_offset=hex2dec('88')  intf_name=''  intf_description=''  timing_constraint=None  locs_specified=off  LOCs={}  io_standard={}  inherit_from_input=off  hdl_port=on  dbl_ovrd=off  block_type=gatewayin
  toDsp_config3 : xbsIndex_r4/Gateway In  gui_display_data_type=Fixed-point  arith_type=Unsigned  n_bits=32  bin_pt=0  preci_type=Single  exp_width=8  frac_width=24  rows=1  columns=1  quantization=Truncate  overflow=Wrap  period=Tclk  UseAsADC=off  ADCChannel='1'  interface=AXI4-Lite  automatic_assignment=off  address_offset=hex2dec('8C')  intf_name=''  intf_description=''  timing_constraint=None  locs_specified=off  LOCs={}  io_standard={}  inherit_from_input=off  hdl_port=on  dbl_ovrd=off  block_type=gatewayin
  toDsp_config4 : xbsIndex_r4/Gateway In  gui_display_data_type=Fixed-point  arith_type=Unsigned  n_bits=32  bin_pt=0  preci_type=Single  exp_width=8  frac_width=24  rows=1  columns=1  quantization=Truncate  overflow=Wrap  period=Tclk  UseAsADC=off  ADCChannel='1'  interface=AXI4-Lite  automatic_assignment=off  address_offset=hex2dec('94')  intf_name=''  intf_description=''  timing_constraint=None  locs_specified=off  LOCs={}  io_standard={}  inherit_from_input=off  hdl_port=on  dbl_ovrd=off  block_type=gatewayin
  toDsp_config5 : xbsIndex_r4/Gateway In  gui_display_data_type=Fixed-point  arith_type=Unsigned  n_bits=32  bin_pt=0  preci_type=Single  exp_width=8  frac_width=24  rows=1  columns=1  quantization=Truncate  overflow=Wrap  period=Tclk  UseAsADC=off  ADCChannel='1'  interface=AXI4-Lite  automatic_assignment=off  address_offset=hex2dec('98')  intf_name=''  intf_description=''  timing_constraint=None  locs_specified=off  LOCs={}  io_standard={}  inherit_from_input=off  hdl_port=on  dbl_ovrd=off  block_type=gatewayin
  toDsp_config6 : xbsIndex_r4/Gateway In  gui_display_data_type=Fixed-point  arith_type=Unsigned  n_bits=32  bin_pt=0  preci_type=Single  exp_width=8  frac_width=24  rows=1  columns=1  quantization=Truncate  overflow=Wrap  period=Tclk  UseAsADC=off  ADCChannel='1'  interface=AXI4-Lite  automatic_assignment=off  address_offset=hex2dec('9C')  intf_name=''  intf_description=''  timing_constraint=None  locs_specified=off  LOCs={}  io_standard={}  inherit_from_input=off  hdl_port=on  dbl_ovrd=off  block_type=gatewayin
  toDsp_config7 : xbsIndex_r4/Gateway In  gui_display_data_type=Fixed-point  arith_type=Unsigned  n_bits=32  bin_pt=0  preci_type=Single  exp_width=8  frac_width=24  rows=1  columns=1  quantization=Truncate  overflow=Wrap  period=Tclk  UseAsADC=off  ADCChannel='1'  interface=AXI4-Lite  automatic_assignment=off  address_offset=hex2dec('A0')  intf_name=''  intf_description=''  timing_constraint=None  locs_specified=off  LOCs={}  io_standard={}  inherit_from_input=off  hdl_port=on  dbl_ovrd=off  block_type=gatewayin
  toDsp_config8 : xbsIndex_r4/Gateway In  gui_display_data_type=Fixed-point  arith_type=Unsigned  n_bits=32  bin_pt=0  preci_type=Single  exp_width=8  frac_width=24  rows=1  columns=1  quantization=Truncate  overflow=Wrap  period=Tclk  UseAsADC=off  ADCChannel='1'  interface=AXI4-Lite  automatic_assignment=off  address_offset=hex2dec('A4')  intf_name=''  intf_description=''  timing_constraint=None  locs_specified=off  LOCs={}  io_standard={}  inherit_from_input=off  hdl_port=on  dbl_ovrd=off  block_type=gatewayin
  Out1 : Outport
  Out2 : Outport  Port=2
  Out3 : Outport  Port=3
  Out4 : Outport  Port=4
  Out5 : Outport  Port=5
  tag scope: Ampl0=global, Ampl1=global, ConfigReg0=global, DDCLOtrack=global, F0=global, F1=global, FBlimit=global, FBreset=global, NotchSimEn=global, RFen=global, RefSource=global, dFsb=global, whiteNoiseGen=global
  wires:
  In1/1 -> toDsp_config0/1
  toDsp_config0/1 -> Register2/1
  fromDsp_status0/1 -> Out1/1
  In2/1 -> toDsp_config1/1
  toDsp_config1/1 -> Register3/1
  fromDsp_status1/1 -> Out2/1
  In3/1 -> toDsp_config2/1
  toDsp_config2/1 -> Register4/1
  fromDsp_status2/1 -> Out3/1
  In4/1 -> toDsp_config3/1
  toDsp_config3/1 -> Register5/1
  fromDsp_status3/1 -> Out4/1
  In5/1 -> toDsp_cmd0/1
  toDsp_cmd0/1 -> Register6/1
  Register3/1 -> Slice6/1, Slice5/1, fromDsp_status1/1
  Register5/1 -> Slice8/1, Slice7/1, fromDsp_status3/1
  Register6/1 -> Slice4/1, Gateway Out1/1
  Slice5/1 -> Reinterpret/1
  Slice6/1 -> Reinterpret1/1
  Register4/1 -> BitBasher4/1, BitBasher3/1, fromDsp_status2/1
  BitBasher3/1 -> Reinterpret2/1
  BitBasher4/1 -> Reinterpret3/1
  Slice7/1 -> Reinterpret4/1
  Slice8/1 -> Reinterpret5/1
  Register2/1 -> fromDsp_status0/1, Slice/1, Slice1/1, Slice2/1, Slice3/1, Slice9/1, Gateway Out6/1, [ConfigReg0]
  Slice1/1 -> [RefSource]
  Slice/1 -> [RFen]
  Slice2/1 -> [NotchSimEn]
  Slice3/1 -> [whiteNoiseGen]
  Reinterpret/1 -> [Ampl0]
  Reinterpret1/1 -> [Ampl1]
  Gateway Out6/1 -> Control Reg/1
  In6/1 -> toDsp_config4/1
  toDsp_config4/1 -> Register1/1
  In7/1 -> toDsp_config5/1
  toDsp_config5/1 -> Register7/1
  In8/1 -> toDsp_config6/1
  toDsp_config6/1 -> Register8/1
  In9/1 -> toDsp_config7/1
  toDsp_config7/1 -> Register9/1
  In10/1 -> toDsp_config8/1
  toDsp_config8/1 -> Register10/1
  Register1/1 -> fromDsp_status4/1
  Register10/1 -> Terminator/1
  Gateway Out/1 -> F0/1
  Slice4/1 -> [FBreset]
  Reinterpret3/1 -> [dFsb]
  Reinterpret2/1 -> [FBlimit]
  Reinterpret5/1 -> [F1]
  Reinterpret4/1 -> Gateway Out/1, [F0]
  Gateway Out1/1 -> Out5/1
  [FBreset] -> Terminator3/1
  [NotchSimEn] -> Terminator2/1
  [F1] -> Terminator1/1
  fromDsp_status4/1 -> Terminator4/1
  Register9/1 -> Terminator5/1
  fromDsp_status7/1 -> Terminator9/1
  fromDsp_status6/1 -> Terminator8/1
  Register8/1 -> Terminator6/1
  Register7/1 -> Terminator7/1
  [Freq] -> fromDsp_status6/1
  [deltaF] -> fromDsp_status5/1
  fromDsp_status5/1 -> Terminator10/1
  Constant/1 -> fromDsp_status7/1
  Slice9/1 -> [DDCLOtrack]

== system CryoDet6/DspCore/DAC demux clock ==
  note: Use DAC clock to generate edge to synchronize simulation of DAC demuxing in FPGA VHDL wrapper
      | output 1 = I
      | 0 = Q
  In1 : Inport
  Add : Sum
  Clock Enable Probe : xbsIndex_r4/Clock Enable Probe  inherit_constraints=on  block_type=ceprobe
      settings: infoedit="Clock enable extractor.  Produces a Boolean output that mirrors the hardware clock enable associated with the input sample rate.<br><br>Hardware notes: in hardware this block costs nothing."
  Constant : Constant  Value=2
  Down Sample : xbsIndex_r4/Down Sample  sample_ratio=2  sample_phase="Last Value of Frame  (most efficient)"  en=off  rst=off  latency=1  dbl_ovrd=off  block_type=dsamp
  Math Function : Math  Operator=mod  SaturateOnIntegerOverflow=on
  Transport Delay : TransportDelay  DelayTime=Tclk/2
  fromdsp_dacdata1_2 : xbsIndex_r4/Gateway Out  inherit_from_input=off  hdl_port=off  rows=1  columns=1  UseAsDAC=off  DACChannel='1'  interface=None  automatic_assignment=on  address_offset=hex2dec('00')  intf_name=''  intf_description=''  timing_constraint=None  locs_specified=off  LOCs={}  io_standard={}  block_type=gatewayout
  IQtoggle : Outport
  wires:
  Clock Enable Probe/1 -> fromdsp_dacdata1_2/1
  Down Sample/1 -> Clock Enable Probe/1
  In1/1 -> Down Sample/1
  fromdsp_dacdata1_2/1 -> Add/1, Transport Delay/1
  Transport Delay/1 -> Add/2
  Add/1 -> Math Function/1
  Math Function/1 -> IQtoggle/1
  Constant/1 -> Math Function/2

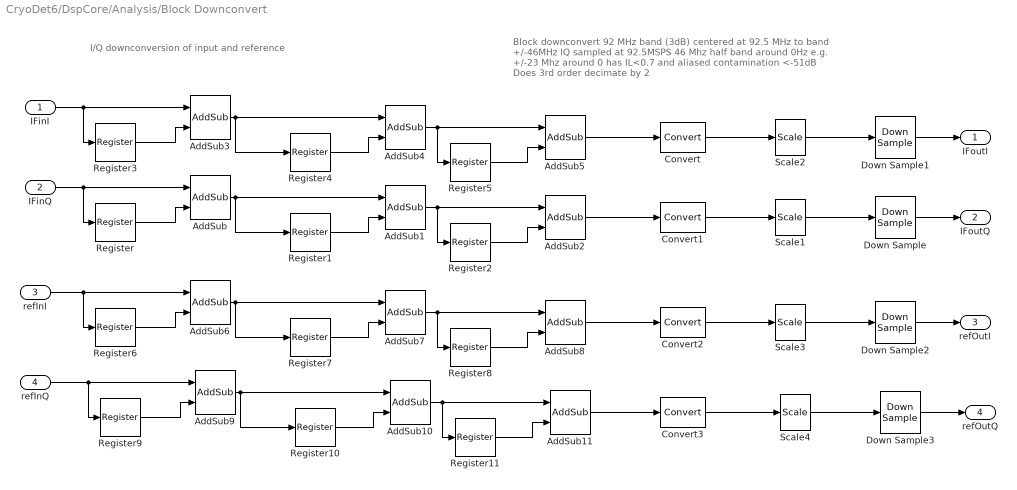
== system CryoDet6/DspCore/Analysis/Block Downconvert ==
  note: I/Q downconversion of input and reference
  note: Block downconvert 92 MHz band (3dB) centered at 92.5 MHz
      | to band +/-46MHz IQ sampled at 92.5MSPS
      | 46 Mhz half band around 0Hz e.g. +/-23 Mhz around 0
      | has IL<0.7 and aliased contamination <-51dB
      | Does 3rd order decimate by 2
  IFinI : Inport
  IFinQ : Inport  Port=2
  refInI : Inport  Port=3
  refInQ : Inport  Port=4
  AddSub{,3,6,9} (4 alike) : xbsIndex_r4/AddSub  mode=Subtraction  use_carryin=off  use_carryout=off  en=off  latency=1  precision=User Defined  arith_type="Signed  (2's comp)"  n_bits=17  bin_pt=15  quantization=Truncate  overflow=Wrap  use_behavioral_HDL=off  hw_selection=Fabric  pipelined=off  dbl_ovrd=off  block_type=addsub
  AddSub{1,4,7,10} (4 alike) : xbsIndex_r4/AddSub  mode=Subtraction  use_carryin=off  use_carryout=off  en=off  latency=1  precision=User Defined  arith_type="Signed  (2's comp)"  n_bits=18  bin_pt=15  quantization=Truncate  overflow=Wrap  use_behavioral_HDL=off  hw_selection=Fabric  pipelined=off  dbl_ovrd=off  block_type=addsub
  AddSub{2,5,8,11} (4 alike) : xbsIndex_r4/AddSub  mode=Subtraction  use_carryin=off  use_carryout=off  en=off  latency=1  precision=User Defined  arith_type="Signed  (2's comp)"  n_bits=19  bin_pt=12  quantization=Truncate  overflow=Wrap  use_behavioral_HDL=off  hw_selection=Fabric  pipelined=off  dbl_ovrd=off  block_type=addsub
  Convert{,1..3} (4 alike) : xbsIndex_r4/Convert  gui_display_data_type=Fixed-point  arith_type="Signed  (2's comp)"  n_bits=16  bin_pt=12  float_type=Single  exp_bits=8  fraction_bits=24  quantization=Truncate  overflow=Saturate  en=off  latency=1  pipeline=off  dbl_ovrd=off  block_type=convert
  Down Sample{,1..3} (4 alike) : xbsIndex_r4/Down Sample  sample_ratio=2  sample_phase="Last Value of Frame  (most efficient)"  en=off  rst=off  latency=1  dbl_ovrd=off  block_type=dsamp
  Register{,1..11} (12 alike) : xbsIndex_r4/Register  init=0  rst=off  en=off  dbl_ovrd=off  block_type=register
  Scale{1..4} (4 alike) : xbsIndex_r4/Scale  scale_factor=-3  dbl_ovrd=off  block_type=scale
  IFoutI : Outport
  IFoutQ : Outport  Port=2
  refOutI : Outport  Port=3
  refOutQ : Outport  Port=4
  wires:
  AddSub2/1 -> Convert1/1
  Scale1/1 -> Down Sample/1
  IFinQ/1 -> Register/1, AddSub/1
  Register/1 -> AddSub/2
  AddSub/1 -> Register1/1, AddSub1/1
  Register1/1 -> AddSub1/2
  AddSub1/1 -> Register2/1, AddSub2/1
  Register2/1 -> AddSub2/2
  AddSub5/1 -> Convert/1
  Scale2/1 -> Down Sample1/1
  IFinI/1 -> Register3/1, AddSub3/1
  Register3/1 -> AddSub3/2
  AddSub3/1 -> Register4/1, AddSub4/1
  Register4/1 -> AddSub4/2
  AddSub4/1 -> Register5/1, AddSub5/1
  Register5/1 -> AddSub5/2
  Down Sample1/1 -> IFoutI/1
  AddSub8/1 -> Convert2/1
  Scale3/1 -> Down Sample2/1
  refInI/1 -> Register6/1, AddSub6/1
  Register6/1 -> AddSub6/2
  AddSub6/1 -> Register7/1, AddSub7/1
  Register7/1 -> AddSub7/2
  AddSub7/1 -> Register8/1, AddSub8/1
  Register8/1 -> AddSub8/2
  Down Sample2/1 -> refOutI/1
  AddSub11/1 -> Convert3/1
  Scale4/1 -> Down Sample3/1
  refInQ/1 -> Register9/1, AddSub9/1
  Register9/1 -> AddSub9/2
  AddSub9/1 -> Register10/1, AddSub10/1
  Register10/1 -> AddSub10/2
  AddSub10/1 -> Register11/1, AddSub11/1
  Register11/1 -> AddSub11/2
  Down Sample3/1 -> refOutQ/1
  Down Sample/1 -> IFoutQ/1
  Convert/1 -> Scale2/1
  Convert1/1 -> Scale1/1
  Convert2/1 -> Scale3/1
  Convert3/1 -> Scale4/1

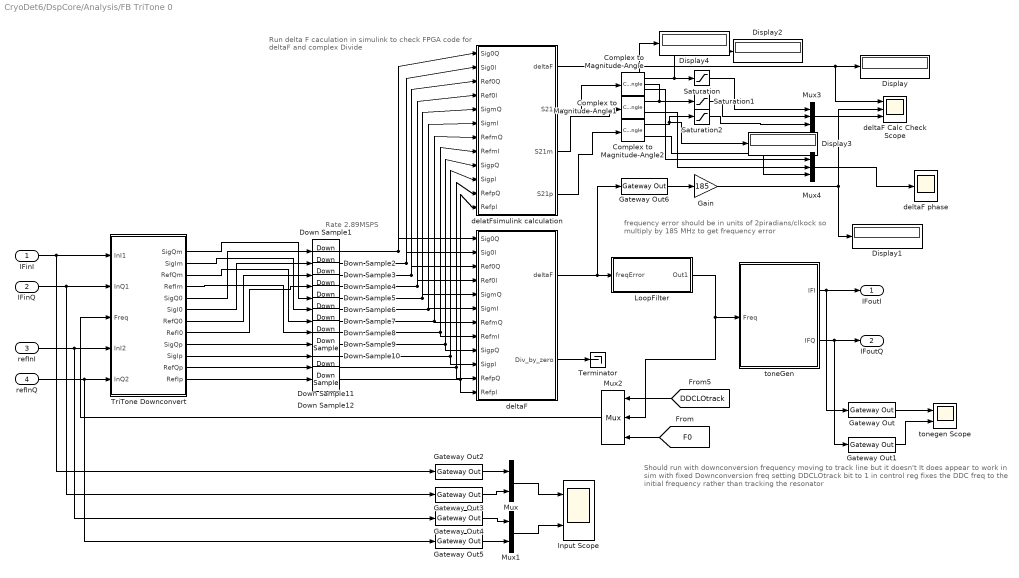
== system CryoDet6/DspCore/Analysis/FB TriTone 0 ==
  note: Rate 2.89MSPS
  note: frequency error should be in units of 2piradians/clkock
      | so multiply by 185 MHz to get frequency error
  note: Run delta F caculation in simulink to check FPGA code
      | for deltaF and complex Divide
  note: Should run with downconversion frequency moving to track line
      | but it doesn't
      | It does appear to work in sim with fixed Downconversion freq
      | setting DDCLOtrack bit to 1 in control reg fixes the DDC freq to the initial frequency rather than tracking the resonator
  IFinI : Inport
  IFinQ : Inport  Port=2
  refInI : Inport  Port=3
  refInQ : Inport  Port=4
  Complex to Magnitude-Angle : ComplexToMagnitudeAngle
  Complex to Magnitude-Angle1 : ComplexToMagnitudeAngle
  Complex to Magnitude-Angle2 : ComplexToMagnitudeAngle
  Display{,1..4} (5 alike) : Display
  Down Sample{1..12} (12 alike) : xbsIndex_r4/Down Sample  sample_ratio=4  sample_phase="Last Value of Frame  (most efficient)"  en=off  rst=off  latency=1  dbl_ovrd=off  block_type=dsamp
  Gain : Gain  Gain=185
  Gateway Out{,1..6} (7 alike) : xbsIndex_r4/Gateway Out  inherit_from_input=off  hdl_port=off  rows=1  columns=1  UseAsDAC=off  DACChannel='1'  interface=None  automatic_assignment=on  address_offset=hex2dec('00')  intf_name=''  intf_description=''  timing_constraint=None  locs_specified=off  LOCs={}  io_standard={}  block_type=gatewayout
  Input Scope : Scope  NumInputPorts=2
      settings: TimeRange=2e-05  YMin=-0.75~-1  YMax=0.75~1  SaveName=ScopeData11
  LoopFilter : Subsystem
  Mux : Mux  Inputs=2
  Mux1 : Mux  Inputs=2
  Mux2 : xbsIndex_r4/Mux  inputs=2  en=off  latency=1  precision=Full  arith_type=Unsigned  n_bits=16  bin_pt=14  quantization=Truncate  overflow=Wrap  dbl_ovrd=off  block_type=mux
  Mux3 : Mux  Inputs=3
  Mux4 : Mux  Inputs=3
  Saturation : Saturate  UpperLimit=2  LowerLimit=-2
  Saturation1 : Saturate  UpperLimit=2  LowerLimit=-2
  Saturation2 : Saturate  UpperLimit=2  LowerLimit=-2
  Terminator : Terminator
  TriTone Downconvert : Subsystem
  delatFsimulink calculation : Subsystem
  deltaF : Subsystem
  deltaF Calc Check Scope : Scope  NumInputPorts=3
      settings: TimeRange=0.001  YMin=-0.2~-0.0106~0.6  YMax=0.35~-0.0096~2  SaveName=ScopeData19  Decimation=16
  deltaF phase : Scope
      settings: TimeRange=0.001  YMin=-3.5  YMax=3  SaveName=ScopeData20  Decimation=16
  toneGen : Subsystem
  tonegen Scope : Scope  NumInputPorts=2
      settings: TimeRange=2e-05  YMin=-0.5~-0.5  YMax=0.5~0.5
  IFoutI : Outport
  IFoutQ : Outport  Port=2
  wires:
  toneGen/2(IFQ) -> IFoutQ/1, Gateway Out1/1
  deltaF/1(deltaF) -> Gateway Out6/1, LoopFilter/1(freqError)
  Gateway Out1/1 -> tonegen Scope/2
  Gateway Out/1 -> tonegen Scope/1
  toneGen/1(IFI) -> IFoutI/1, Gateway Out/1
  TriTone Downconvert/9(SigQp) -> Down Sample9/1
  TriTone Downconvert/10(SigIp) -> Down Sample10/1
  TriTone Downconvert/11(RefQp) -> Down Sample11/1
  TriTone Downconvert/12(RefIp) -> Down Sample12/1
  IFinI/1 -> Gateway Out2/1, TriTone Downconvert/1(InI1)
  IFinQ/1 -> Gateway Out3/1, TriTone Downconvert/2(InQ1)
  refInQ/1 -> Gateway Out5/1, TriTone Downconvert/5(InQ2)
  refInI/1 -> Gateway Out4/1, TriTone Downconvert/4(InI2)
  Gateway Out2/1 -> Mux/1
  Gateway Out3/1 -> Mux/2
  Gateway Out4/1 -> Mux1/1
  Gateway Out5/1 -> Mux1/2
  Mux/1 -> Input Scope/1
  Mux1/1 -> Input Scope/2
  LoopFilter/1(Out1) -> Mux2/2, toneGen/1(Freq)
  [F0] -> Mux2/3
  Mux2/1 -> TriTone Downconvert/3(Freq)
  [DDCLOtrack] -> Mux2/1
  deltaF/2(Div_by_zero) -> Terminator/1
  Gateway Out6/1 -> Gain/1
  delatFsimulink calculation/1(deltaF) -> deltaF Calc Check Scope/1, Display/1
  Gain/1 -> Display1/1, deltaF Calc Check Scope/2
  Down Sample1/1 -> delatFsimulink calculation/1(Sig0Q), deltaF/1(Sig0Q)
  Down Sample2/1 -> delatFsimulink calculation/2(Sig0I), deltaF/2(Sig0I)
  Down Sample3/1 -> delatFsimulink calculation/3(Ref0Q), deltaF/3(Ref0Q)
  Down Sample4/1 -> delatFsimulink calculation/4(Ref0I), deltaF/4(Ref0I)
  Down Sample5/1 -> delatFsimulink calculation/5(SigmQ), deltaF/5(SigmQ)
  Down Sample6/1 -> delatFsimulink calculation/6(SigmI), deltaF/6(SigmI)
  Down Sample7/1 -> delatFsimulink calculation/7(RefmQ), deltaF/7(RefmQ)
  Down Sample8/1 -> delatFsimulink calculation/8(RefmI), deltaF/8(RefmI)
  Down Sample9/1 -> delatFsimulink calculation/9(SigpQ), deltaF/9(SigpQ)
  Down Sample10/1 -> delatFsimulink calculation/10(SigpI), deltaF/10(SigpI)
  Down Sample11/1 -> delatFsimulink calculation/11(RefpQ), deltaF/11(RefpQ)
  Down Sample12/1 -> delatFsimulink calculation/12(RefpI), deltaF/12(RefpI)
  Mux3/1 -> deltaF Calc Check Scope/3
  delatFsimulink calculation/2(S21) -> Complex to Magnitude-Angle/1
  delatFsimulink calculation/3(S21m) -> Complex to Magnitude-Angle1/1
  delatFsimulink calculation/4(S21p) -> Complex to Magnitude-Angle2/1
  Complex to Magnitude-Angle/1 -> Display2/1, Saturation/1
  Complex to Magnitude-Angle1/1 -> Display4/1, Saturation1/1
  Complex to Magnitude-Angle2/1 -> Display3/1, Saturation2/1
  Saturation/1 -> Mux3/1
  Saturation1/1 -> Mux3/2
  Saturation2/1 -> Mux3/3
  Complex to Magnitude-Angle/2 -> Mux4/1
  Complex to Magnitude-Angle1/2 -> Mux4/2
  Complex to Magnitude-Angle2/2 -> Mux4/3
  Mux4/1 -> deltaF phase/1
  TriTone Downconvert/1(SigQm) -> Down Sample5/1
  TriTone Downconvert/2(SigIm) -> Down Sample6/1
  TriTone Downconvert/3(RefQm) -> Down Sample7/1
  TriTone Downconvert/4(RefIm) -> Down Sample8/1
  TriTone Downconvert/8(RefI0) -> Down Sample4/1
  TriTone Downconvert/7(RefQ0) -> Down Sample3/1
  TriTone Downconvert/6(SigI0) -> Down Sample2/1
  TriTone Downconvert/5(SigQ0) -> Down Sample1/1

== system CryoDet6/DspCore/Analysis/FB TriTone 1 ==
  note: Dummy for now
      | Copy from first channel when that one works
  IFinI : Inport
  IFinQ : Inport  Port=2
  refInI : Inport  Port=3
  refInQ : Inport  Port=4
  Constant : xbsIndex_r4/Constant  const=0  gui_display_data_type=Fixed-point  arith_type=Signed (2's comp)  n_bits=16  bin_pt=15  preci_type=Single  exp_width=8  frac_width=24  explicit_period=off  period=1  equ=P=C  opselect=C  inp2=PCIN>>17  opr=+  inp1=P  carry=CIN  dbl_ovrd=off  block_type=constant
  Terminator{,1..3} (4 alike) : Terminator
  IFoutI : Outport
  IFoutQ : Outport  Port=2
  wires:
  Constant/1 -> IFoutQ/1, IFoutI/1
  IFinQ/1 -> Terminator/1
  refInI/1 -> Terminator3/1
  refInQ/1 -> Terminator2/1
  IFinI/1 -> Terminator1/1
